simulink model "torqueWalkingMultipleStateCoefficientR2017b"  (Simulink 9.0)
settings: Solver=FixedStepDiscrete  StartTime=0.0  StopTime=Config.t_end  FixedStep=Config.t_step  RelTol=1e-3  EnableMultiTasking=on
InitFcn:
  | cd(fileparts(which(bdroot)));
  | initTorqueWalkingParamInScheme;
StopFcn:
  | cd(fileparts(which(bdroot)));
  | disp_early_termination
undefined symbols (not defined in the file or in its folder): biasVectorConstraint_feet, Config, CONFIG, ConstraintMatrix_feet, DiscIntNeverNeededParam, Gains, ROBOT_DOF, Sat
libraries: WBToolboxLibrary x113, commchan3 x2, simulink x2
(part 2 of 4)

== system torqueWalkingMultipleStateCoefficientR2017b/Robot State and References/Smooth References  ==
  state : Inport
  references_LFoot : Inport  Port=2
  references_RFoot : Inport  Port=3
  references_CoM : Inport  Port=4
  references_rot_task : Inport  Port=5
  references_LHand : Inport  Port=6
  references_RHand : Inport  Port=7
  references_s : Inport  Port=8
  Choose Smoothed or Direct References : Subsystem
  Selector{1..3,5..6} (5 alike) : Selector  NumberOfDimensions=2  InputPortWidth=3  IndexOptions=Index vector (dialog),Index vector (dialog)  Indices=[1:3],1  OutputSizes=1,1
  Selector{8..11} (4 alike) : Selector  NumberOfDimensions=2  InputPortWidth=3  IndexOptions=Index vector (dialog),Index vector (dialog)  Indices=[4:6],[1:3]  OutputSizes=1,1
  Selector4 : Selector  NumberOfDimensions=2  InputPortWidth=3  IndexOptions=Index vector (dialog),Index vector (dialog)  Indices=[1:3],[1:3]  OutputSizes=1,1
  Selector7 : Selector  NumberOfDimensions=2  InputPortWidth=ROBOT_DOF  IndexOptions=Index vector (dialog),Index vector (dialog)  Indices=[1:ROBOT_DOF],1  OutputSizes=1,1
  Smooth Reference Orientations : Subsystem
  Smooth Reference Positions : Subsystem
  pos_vel_acc_CoM_des : Outport
  pose_vel_acc_LFoot_des : Outport  Port=2
  pose_vel_acc_RFoot_des : Outport  Port=3
  orient_vel_acc_rot_task_des : Outport  Port=4
  pose_vel_acc_LHand_des : Outport  Port=5
  pose_vel_acc_RHand_des : Outport  Port=6
  s_sDot_sDDot_ref : Outport  Port=7
  wires:
  references_CoM/1 -> Choose Smoothed or Direct References/7(references_CoM), Selector1/1
  Selector1/1 -> Smooth Reference Positions/1(pos_CoM_des)
  references_LFoot/1 -> Choose Smoothed or Direct References/8(references_LFoot), Selector9/1, Selector2/1
  Selector2/1 -> Smooth Reference Positions/2(pos_LFoot_des)
  references_RFoot/1 -> Selector8/1, Choose Smoothed or Direct References/9(references_RFoot), Selector6/1
  Selector6/1 -> Smooth Reference Positions/3(pos_RFoot_des)
  references_s/1 -> Selector7/1, Choose Smoothed or Direct References/12(references_s)
  Selector7/1 -> Smooth Reference Positions/4(s_des)
  references_rot_task/1 -> Selector4/1, Choose Smoothed or Direct References/13(references_rot_task)
  Selector4/1 -> Smooth Reference Orientations/3(w_R_Rot_task_des)
  Selector8/1 -> Smooth Reference Orientations/2(w_R_RFoot_des)
  Selector9/1 -> Smooth Reference Orientations/1(w_R_LFoot_des)
  Smooth Reference Positions/1(smooth_references_CoM) -> Choose Smoothed or Direct References/1(smooth_references_CoM)
  Smooth Reference Orientations/3(smooth_orient_vel_acc_Rot_task) -> Choose Smoothed or Direct References/16(smooth_references_rot_task)
  Smooth Reference Orientations/2(smooth_orient_vel_acc_RFoot) -> Choose Smoothed or Direct References/15(smooth_orient_vel_acc_RFoot)
  Smooth Reference Orientations/1(smooth_orient_vel_acc_LFoot) -> Choose Smoothed or Direct References/14(smooth_orient_vel_acc_LFoot)
  Choose Smoothed or Direct References/1(pos_vel_acc_CoM_des) -> pos_vel_acc_CoM_des/1
  Choose Smoothed or Direct References/2(pose_vel_acc_LFoot_des) -> pose_vel_acc_LFoot_des/1
  Choose Smoothed or Direct References/7(s_sDot_sDDot_ref) -> s_sDot_sDDot_ref/1
  Choose Smoothed or Direct References/4(orient_vel_acc_rot_task_des) -> orient_vel_acc_rot_task_des/1
  Choose Smoothed or Direct References/3(pose_vel_acc_RFoot_des) -> pose_vel_acc_RFoot_des/1
  state/1 -> Smooth Reference Positions/7(state), Smooth Reference Orientations/6(state)
  Smooth Reference Positions/2(smooth_pos_vel_acc_LFoot) -> Choose Smoothed or Direct References/2(smooth_pos_vel_acc_LFoot)
  Smooth Reference Positions/3(smooth_pos_vel_acc_RFoot) -> Choose Smoothed or Direct References/3(smooth_pos_vel_acc_RFoot)
  Smooth Reference Positions/6(smooth_references_s) -> Choose Smoothed or Direct References/6(smooth_references_s)
  Selector3/1 -> Smooth Reference Positions/5(pos_LHand_des)
  references_LHand/1 -> Selector3/1, Selector11/1, Choose Smoothed or Direct References/10(references_LHand)
  Selector5/1 -> Smooth Reference Positions/6(pos_RHand_des)
  references_RHand/1 -> Selector5/1, Selector10/1, Choose Smoothed or Direct References/11(references_RHand)
  Smooth Reference Positions/4(smooth_pos_vel_acc_LHand) -> Choose Smoothed or Direct References/4(smooth_pos_vel_acc_LHand)
  Smooth Reference Positions/5(smooth_pos_vel_acc_RHand) -> Choose Smoothed or Direct References/5(smooth_pos_vel_acc_RHand)
  Selector11/1 -> Smooth Reference Orientations/4(w_R_LHand_des)
  Selector10/1 -> Smooth Reference Orientations/5(w_R_RHand_des)
  Smooth Reference Orientations/4(smooth_orient_vel_acc_LHand) -> Choose Smoothed or Direct References/17(smooth_orient_vel_acc_LHand)
  Smooth Reference Orientations/5(smooth_orient_vel_acc_RHand) -> Choose Smoothed or Direct References/18(smooth_orient_vel_acc_RHand)
  Choose Smoothed or Direct References/5(pose_vel_acc_LHand_des) -> pose_vel_acc_LHand_des/1
  Choose Smoothed or Direct References/6(pose_vel_acc_RHand_des) -> pose_vel_acc_RHand_des/1

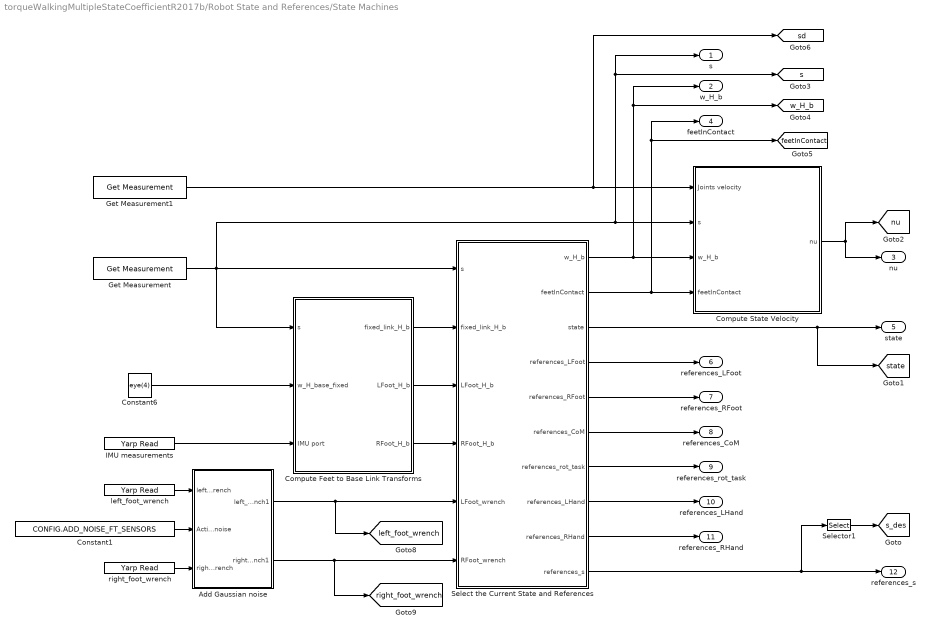
== system torqueWalkingMultipleStateCoefficientR2017b/Robot State and References/State Machines ==
  Add Gaussian noise : Subsystem
  Compute Feet to Base Link Transforms : Subsystem
  Compute State Velocity : Subsystem
  Constant1 : Constant  Value=CONFIG.ADD_NOISE_FT_SENSORS
  Constant6 : Constant  Value=eye(4)
  Get Measurement : WBToolboxLibrary/wholeBodyStates/Get Measurement  measuredType=Joints Position
      settings: SourceProductName=Whole Body Toolbox
  Get Measurement1 : WBToolboxLibrary/wholeBodyStates/Get Measurement  measuredType=Joints Velocity
      settings: SourceProductName=Whole Body Toolbox
  IMU measurements : WBToolboxLibrary/Utilities/Yarp Read  portName=Ports.IMU  signalSize=12  timeout=0.5  blocking=off  timestamp=off  autoconnect=on  errorOnConnection=off
      settings: SourceProductName=Whole Body Toolbox
  Select the Current State and References : Subsystem
  Selector1 : Selector  NumberOfDimensions=2  InputPortWidth=ROBOT_DOF  IndexOptions=Index vector (dialog),Index vector (dialog)  Indices=[1:ROBOT_DOF],1  OutputSizes=1,1
  left_foot_wrench : WBToolboxLibrary/Utilities/Yarp Read  portName=Ports.LEFT_FOOT_EXT_WRENCH  signalSize=6  timeout=0.5  blocking=off  timestamp=off  autoconnect=on  errorOnConnection=on
      settings: SourceProductName=Whole Body Toolbox
  right_foot_wrench : WBToolboxLibrary/Utilities/Yarp Read  portName=Ports.RIGHT_FOOT_EXT_WRENCH  signalSize=6  timeout=0.5  blocking=off  timestamp=off  autoconnect=on  errorOnConnection=on
      settings: SourceProductName=Whole Body Toolbox
  s : Outport
  w_H_b : Outport  Port=2
  nu : Outport  Port=3
  feetInContact : Outport  Port=4
  state : Outport  Port=5
  references_LFoot : Outport  Port=6
  references_RFoot : Outport  Port=7
  references_CoM : Outport  Port=8
  references_rot_task : Outport  Port=9
  references_LHand : Outport  Port=10
  references_RHand : Outport  Port=11
  references_s : Outport  Port=12
  tag scope: feetInContact=global, left_foot_wrench=global, nu=global, right_foot_wrench=global, s=global, s_des=global, sd=global, state=global, w_H_b=global
  wires:
  Get Measurement/1 -> Compute Feet to Base Link Transforms/1(s), Compute State Velocity/2(s), s/1, [s], Select the Current State and References/1(s)
  Constant6/1 -> Compute Feet to Base Link Transforms/2(w_H_base_fixed)
  Compute Feet to Base Link Transforms/1(fixed_link_H_b) -> Select the Current State and References/2(fixed_link_H_b)
  Select the Current State and References/1(w_H_b) -> w_H_b/1, [w_H_b], Compute State Velocity/3(w_H_b)
  Select the Current State and References/2(feetInContact) -> feetInContact/1, [feetInContact], Compute State Velocity/4("feetInContact ")
  Compute State Velocity/1(nu) -> nu/1, [nu]
  Select the Current State and References/3(state) -> [state], state/1
  Select the Current State and References/10(references_s) -> references_s/1, Selector1/1
  Select the Current State and References/6(references_CoM) -> references_CoM/1
  Select the Current State and References/7(references_rot_task) -> references_rot_task/1
  Select the Current State and References/5(references_RFoot) -> references_RFoot/1
  Select the Current State and References/4(references_LFoot) -> references_LFoot/1
  Selector1/1 -> [s_des]
  Compute Feet to Base Link Transforms/2(LFoot_H_b) -> Select the Current State and References/3(LFoot_H_b)
  Compute Feet to Base Link Transforms/3(RFoot_H_b) -> Select the Current State and References/4(RFoot_H_b)
  Select the Current State and References/8(references_LHand) -> references_LHand/1
  Select the Current State and References/9(references_RHand) -> references_RHand/1
  Get Measurement1/1 -> [sd], Compute State Velocity/1(Joints velocity)
  IMU measurements/1 -> Compute Feet to Base Link Transforms/3(IMU port)
  Add Gaussian noise/1(left_foot_wrench1) -> [left_foot_wrench], Select the Current State and References/5(LFoot_wrench)
  Add Gaussian noise/2(right_foot_wrench1) -> [right_foot_wrench], Select the Current State and References/6(RFoot_wrench)
  left_foot_wrench/1 -> Add Gaussian noise/1(left_foot_wrench)
  Constant1/1 -> Add Gaussian noise/2(Activate noise)
  right_foot_wrench/1 -> Add Gaussian noise/3(right_foot_wrench)

== system torqueWalkingMultipleStateCoefficientR2017b/Subsystem/task errors ==
  pos_vel_CoM : Inport
  pos_vel_acc_CoM_des : Inport  Port=2
  orient_vel_rot_rask : Inport  Port=3
  pos_vel_acc_rot_task_des : Inport  Port=4
  pose_vel_LFoot : Inport  Port=5
  pos_vel_acc_LFoot_des : Inport  Port=6
  pose_vel_RFoot : Inport  Port=7
  pos_vel_acc_RFoot_des : Inport  Port=8
  Rotation Error Left Foot : Subsystem
  Rotation Error Left Foot1 : Subsystem
  Rotation Error Rotational Task : Subsystem
  Selector{,2..6} (6 alike) : Selector  NumberOfDimensions=2  InputPortWidth=3  IndexOptions=Index vector (dialog),Index vector (dialog)  Indices=[1:3],1  OutputSizes=1,1
  Selector12 : Selector  NumberOfDimensions=2  InputPortWidth=3  IndexOptions=Index vector (dialog),Index vector (dialog)  Indices=[1:3],[1:3]  OutputSizes=1,1
  Selector13 : Selector  NumberOfDimensions=2  InputPortWidth=3  IndexOptions=Index vector (dialog),Index vector (dialog)  Indices=[1:3],[1:3]  OutputSizes=1,1
  Selector{7..9,15} (4 alike) : Selector  NumberOfDimensions=2  InputPortWidth=3  IndexOptions=Index vector (dialog),Index vector (dialog)  Indices=[4:6],[1:3]  OutputSizes=1,1
  Sum : Sum  Inputs=+-|
  Sum2 : Sum  Inputs=+-|
  Sum3 : Sum  Inputs=+-|
  Vector Concatenate : Concatenate  NumInputs=6
  taskErrors : Outport
  wires:
  Rotation Error Left Foot/1(|1-R^T*RDes|^2) -> Vector Concatenate/4
  Sum3/1 -> Vector Concatenate/5
  Sum2/1 -> Vector Concatenate/3
  Selector6/1 -> Sum3/2
  Selector5/1 -> Sum3/1
  pose_vel_LFoot/1 -> Selector3/1, Selector7/1
  pose_vel_RFoot/1 -> Selector9/1, Selector5/1
  Selector4/1 -> Sum2/2
  Selector/1 -> Sum/1
  Rotation Error Left Foot1/1(|1-R^T*RDes|^2) -> Vector Concatenate/6
  Selector13/1 -> Rotation Error Rotational Task/1(w_R_rot_task)
  Selector12/1 -> Rotation Error Rotational Task/2(w_R_rot_task_des)
  pos_vel_acc_LFoot_des/1 -> Selector15/1, Selector4/1
  Selector15/1 -> Rotation Error Left Foot/2(w_R_RFoot_des)
  Sum/1 -> Vector Concatenate/1
  Rotation Error Rotational Task/1(|1-R^T*RDes|^2) -> Vector Concatenate/2
  Selector8/1 -> Rotation Error Left Foot1/2(w_R_RFoot_des)
  orient_vel_rot_rask/1 -> Selector13/1
  Selector2/1 -> Sum/2
  Selector9/1 -> Rotation Error Left Foot1/1(w_R_RFoot)
  Selector3/1 -> Sum2/1
  pos_vel_acc_rot_task_des/1 -> Selector12/1
  pos_vel_acc_RFoot_des/1 -> Selector8/1, Selector6/1
  pos_vel_CoM/1 -> Selector/1
  Selector7/1 -> Rotation Error Left Foot/1(w_R_RFoot)
  pos_vel_acc_CoM_des/1 -> Selector2/1
  Vector Concatenate/1 -> taskErrors/1

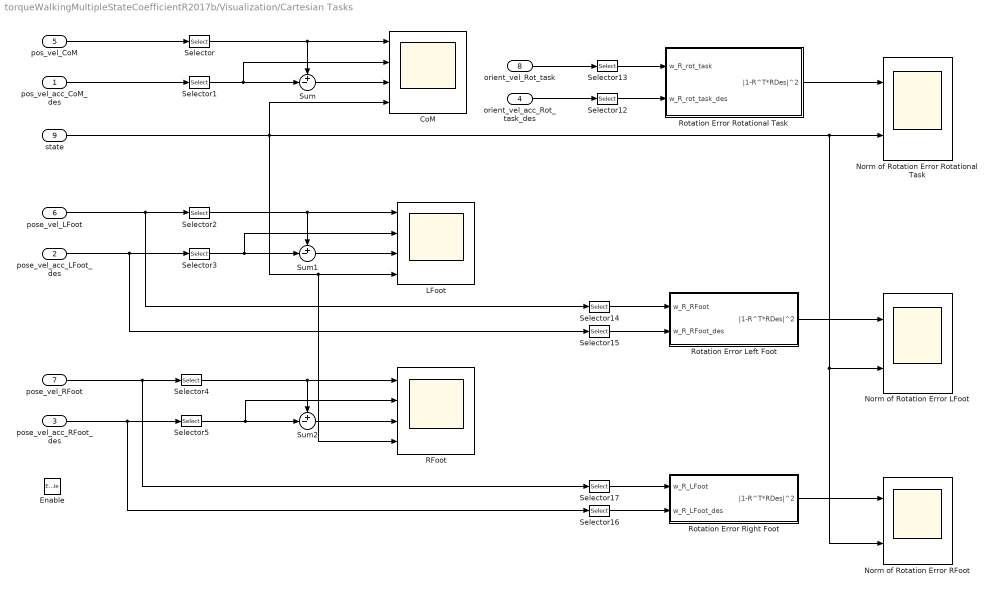
== system torqueWalkingMultipleStateCoefficientR2017b/Visualization/Cartesian Tasks ==
  pos_vel_acc_CoM_des : Inport
  pose_vel_acc_LFoot_des : Inport  Port=2
  pose_vel_acc_RFoot_des : Inport  Port=3
  orient_vel_acc_Rot_task_des : Inport  Port=4
  pos_vel_CoM : Inport  Port=5
  pose_vel_LFoot : Inport  Port=6
  pose_vel_RFoot : Inport  Port=7
  orient_vel_Rot_task : Inport  Port=8
  state : Inport  Port=9
  Enable : EnablePort
  CoM : Scope  NumInputPorts=4
  LFoot : Scope  NumInputPorts=4
  Norm of Rotation Error LFoot : Scope  NumInputPorts=2
  Norm of Rotation Error RFoot : Scope  NumInputPorts=2
  Norm of Rotation Error Rotational Task : Scope  NumInputPorts=2
  RFoot : Scope  NumInputPorts=4
  Rotation Error Left Foot : Subsystem
  Rotation Error Right Foot : Subsystem
  Rotation Error Rotational Task : Subsystem
  Selector{,1..5} (6 alike) : Selector  NumberOfDimensions=2  InputPortWidth=3  IndexOptions=Index vector (dialog),Index vector (dialog)  Indices=[1:3],1  OutputSizes=1,1
  Selector12 : Selector  NumberOfDimensions=2  InputPortWidth=3  IndexOptions=Index vector (dialog),Index vector (dialog)  Indices=[1:3],[1:3]  OutputSizes=1,1
  Selector13 : Selector  NumberOfDimensions=2  InputPortWidth=3  IndexOptions=Index vector (dialog),Index vector (dialog)  Indices=[1:3],[1:3]  OutputSizes=1,1
  Selector{14..17} (4 alike) : Selector  NumberOfDimensions=2  InputPortWidth=3  IndexOptions=Index vector (dialog),Index vector (dialog)  Indices=[4:6],[1:3]  OutputSizes=1,1
  Sum : Sum  Inputs=+-|
  Sum1 : Sum  Inputs=+-|
  Sum2 : Sum  Inputs=+-|
  wires:
  Selector1/1 -> CoM/2, Sum/2
  pos_vel_CoM/1 -> Selector/1
  pos_vel_acc_CoM_des/1 -> Selector1/1
  Selector2/1 -> Sum1/1, LFoot/1
  Selector3/1 -> Sum1/2, LFoot/2
  Selector4/1 -> Sum2/1, RFoot/1
  Selector5/1 -> RFoot/2, Sum2/2
  pose_vel_RFoot/1 -> Selector4/1, Selector17/1
  state/1 -> Norm of Rotation Error RFoot/2, Norm of Rotation Error LFoot/2, Norm of Rotation Error Rotational Task/2, CoM/4, RFoot/4, LFoot/4
  pose_vel_acc_RFoot_des/1 -> Selector5/1, Selector16/1
  pose_vel_LFoot/1 -> Selector2/1, Selector14/1
  Selector12/1 -> Rotation Error Rotational Task/2(w_R_rot_task_des)
  pose_vel_acc_LFoot_des/1 -> Selector15/1, Selector3/1
  orient_vel_acc_Rot_task_des/1 -> Selector12/1
  orient_vel_Rot_task/1 -> Selector13/1
  Selector/1 -> Sum/1, CoM/1
  Sum/1 -> CoM/3
  Sum1/1 -> LFoot/3
  Sum2/1 -> RFoot/3
  Rotation Error Rotational Task/1(|1-R^T*RDes|^2) -> Norm of Rotation Error Rotational Task/1
  Selector13/1 -> Rotation Error Rotational Task/1(w_R_rot_task)
  Rotation Error Left Foot/1(|1-R^T*RDes|^2) -> Norm of Rotation Error LFoot/1
  Selector14/1 -> Rotation Error Left Foot/1(w_R_RFoot)
  Selector15/1 -> Rotation Error Left Foot/2(w_R_RFoot_des)
  Rotation Error Right Foot/1(|1-R^T*RDes|^2) -> Norm of Rotation Error RFoot/1
  Selector16/1 -> Rotation Error Right Foot/2(w_R_LFoot_des)
  Selector17/1 -> Rotation Error Right Foot/1(w_R_LFoot)

== system torqueWalkingMultipleStateCoefficientR2017b/Visualization/Emergency Stop ==
  note: Stop the simulation when the force on each feet is below a threshold (i.e. robot falls)
  F_l_foot : Inport
  F_r_foot : Inport  Port=2
  Enable : EnablePort
  Compare To Constant : simulink/Logic and Bit Operations/Compare To Constant  relop=<=  const=50  OutDataTypeStr=boolean
  Compare To Constant1 : simulink/Logic and Bit Operations/Compare To Constant  relop=<=  const=50  OutDataTypeStr=boolean
  Constant3 : Constant  Value=0  OutDataTypeStr=boolean
  Constant4 : Constant  OutDataTypeStr=boolean
  Logical Operator : Logic  AllPortsSameDT=off  OutDataTypeStr=boolean
  Stop Simulation : Stop
  Switch1 : Switch  Criteria=u2 ~= 0  Threshold=0.5
  To Workspace : ToWorkspace  VariableName=no_force_on_feet  SaveFormat=Timeseries  SampleTime=-1
      settings: MaxDataPoints=1
  select_pose5 : Selector  InputPortWidth=6  IndexOptions=Index vector (dialog)  Indices=[3]  OutputSizes=1
  select_pose6 : Selector  InputPortWidth=6  IndexOptions=Index vector (dialog)  Indices=[3]  OutputSizes=1
  wires:
  F_l_foot/1 -> select_pose5/1
  F_r_foot/1 -> select_pose6/1
  Compare To Constant/1 -> Logical Operator/1
  Compare To Constant1/1 -> Logical Operator/2
  Logical Operator/1 -> Switch1/2
  Switch1/1 -> To Workspace/1, Stop Simulation/1
  Constant4/1 -> Switch1/1
  Constant3/1 -> Switch1/3
  select_pose5/1 -> Compare To Constant/1
  select_pose6/1 -> Compare To Constant1/1

== system torqueWalkingMultipleStateCoefficientR2017b/Visualization/Emergency Stop1 ==
  exitFlagQP : Inport
  Enable : EnablePort
  Constant : Constant  Value=2
  Constant1 : Constant  Value=0  OutDataTypeStr=boolean
  Constant2 : Constant  OutDataTypeStr=boolean
  Stop Simulation : Stop
  Sum : Sum  Inputs=|++
  Switch : Switch  Criteria=u2 > Threshold  Threshold=0.1
  To Workspace : ToWorkspace  VariableName=exitFlagQP_unsuccessful  SaveFormat=Timeseries  SampleTime=-1
      settings: MaxDataPoints=1
  wires:
  exitFlagQP/1 -> Sum/1
  Sum/1 -> Switch/2
  Constant/1 -> Sum/2
  Constant1/1 -> Switch/1
  Constant2/1 -> Switch/3
  Switch/1 -> To Workspace/1, Stop Simulation/1

== system torqueWalkingMultipleStateCoefficientR2017b/Visualization/Emergency Stop2 ==
  note: Stop the simulation when the ZMP goes out of the support polygon
  ZMP : Inport
  support_polygon : Inport  Port=2
  Enable : EnablePort
  Constant3 : Constant  Value=0  OutDataTypeStr=boolean
  Constant4 : Constant  OutDataTypeStr=boolean
  Logical Operator : Logic  Operator=OR  AllPortsSameDT=off  OutDataTypeStr=boolean
  Logical Operator1 : Logic  Operator=OR  AllPortsSameDT=off  OutDataTypeStr=boolean
  Logical Operator2 : Logic  Operator=OR  AllPortsSameDT=off  OutDataTypeStr=boolean
  Logical Operator3 : Logic  Inputs=3  AllPortsSameDT=off  OutDataTypeStr=boolean
  Memory{,1..3} (4 alike) : Memory
  Relational Operator : RelationalOperator  Operator=<  OutDataTypeStr=boolean  RndMeth=Simplest
  Relational Operator1 : RelationalOperator  Operator=>  OutDataTypeStr=boolean  RndMeth=Simplest
  Relational Operator2 : RelationalOperator  Operator=<  OutDataTypeStr=boolean  RndMeth=Simplest
  Relational Operator3 : RelationalOperator  Operator=>  OutDataTypeStr=boolean  RndMeth=Simplest
  Relational Operator4 : RelationalOperator  Operator=<  OutDataTypeStr=boolean  RndMeth=Simplest
  Relational Operator5 : RelationalOperator  Operator=>  OutDataTypeStr=boolean  RndMeth=Simplest
  Stop Simulation : Stop
  Sum of Elements : Sum  Inputs=+
  Switch1 : Switch  Criteria=u2 ~= 0  Threshold=0.5
  To Workspace : ToWorkspace  VariableName=ZMP_out_of_bounds  SaveFormat=Timeseries  SampleTime=-1
      settings: MaxDataPoints=1
  select_pose1 : Selector  NumberOfDimensions=2  InputPortWidth=6  IndexOptions=Index vector (dialog),Index vector (dialog)  Indices=[1 2],2  OutputSizes=1,1
  select_pose2 : Selector  NumberOfDimensions=2  InputPortWidth=6  IndexOptions=Index vector (dialog),Index vector (dialog)  Indices=[1 2],2  OutputSizes=1,1
  select_pose3 : Selector  NumberOfDimensions=2  InputPortWidth=6  IndexOptions=Index vector (dialog),Index vector (dialog)  Indices=[1 2],1  OutputSizes=1,1
  select_pose4 : Selector  NumberOfDimensions=2  InputPortWidth=6  IndexOptions=Index vector (dialog),Index vector (dialog)  Indices=[1 2],2  OutputSizes=1,1
  select_pose5 : Selector  NumberOfDimensions=2  InputPortWidth=6  IndexOptions=Index vector (dialog),Index vector (dialog)  Indices=[1 2],1  OutputSizes=1,1
  select_pose6 : Selector  NumberOfDimensions=2  InputPortWidth=6  IndexOptions=Index vector (dialog),Index vector (dialog)  Indices=[1 2],1  OutputSizes=1,1
  wires:
  Constant3/1 -> Switch1/3
  Constant4/1 -> Switch1/1
  Switch1/1 -> To Workspace/1, Stop Simulation/1
  Sum of Elements/1 -> Switch1/2
  select_pose6/1 -> Relational Operator/2
  select_pose1/1 -> Relational Operator1/2
  Relational Operator/1 -> Logical Operator/1
  Relational Operator1/1 -> Logical Operator/2
  Logical Operator/1 -> Logical Operator3/1
  support_polygon/1 -> Memory/1, select_pose1/1, select_pose6/1
  ZMP/1 -> Memory1/1, Relational Operator1/1, Relational Operator/1
  Logical Operator1/1 -> Logical Operator3/2
  select_pose3/1 -> Relational Operator2/2
  Relational Operator3/1 -> Logical Operator1/2
  Relational Operator2/1 -> Logical Operator1/1
  select_pose2/1 -> Relational Operator3/2
  Memory/1 -> Memory2/1, select_pose2/1, select_pose3/1
  Memory2/1 -> select_pose4/1, select_pose5/1
  Memory3/1 -> Relational Operator5/1, Relational Operator4/1
  select_pose4/1 -> Relational Operator5/2
  Memory1/1 -> Memory3/1, Relational Operator3/1, Relational Operator2/1
  select_pose5/1 -> Relational Operator4/2
  Relational Operator4/1 -> Logical Operator2/1
  Relational Operator5/1 -> Logical Operator2/2
  Logical Operator2/1 -> Logical Operator3/3
  Logical Operator3/1 -> Sum of Elements/1

== system torqueWalkingMultipleStateCoefficientR2017b/Visualization/External wrench  applied ==
  Constant : Constant  Value=CONFIG.APPLY_EXTERNAL_WRENCH
  don't check ZMP : Outport
  wires:
  Constant/1 -> don't check ZMP/1

== system torqueWalkingMultipleStateCoefficientR2017b/Visualization/Forces and Torques ==
  tau measured : Inport
  tau desired : Inport  Port=2
  f LFoot desired : Inport  Port=3
  f RFoot desired : Inport  Port=4
  exitFlag QP : Inport  Port=5
  f LFoot : Inport  Port=6
  f RFoot : Inport  Port=7
  state : Inport  Port=8
  Enable : EnablePort
  Demux{1..4} (4 alike) : Demux  Outputs=[3;3]
  DoFs converter : WBToolboxLibrary/Utilities/DoFs converter  yarp2WBIOption=From YARP to WBI
      settings: SourceProductName=Whole Body Toolbox
  DoFs converter1 : WBToolboxLibrary/Utilities/DoFs converter  yarp2WBIOption=From YARP to WBI
      settings: SourceProductName=Whole Body Toolbox
  DoFs converter2 : WBToolboxLibrary/Utilities/DoFs converter  yarp2WBIOption=From YARP to WBI
      settings: SourceProductName=Whole Body Toolbox
  QP status : Scope  NumInputPorts=2
  Sum : Sum  Inputs=+-|
  Sum1 : Sum  Inputs=|+-
  Sum2 : Sum  Inputs=+-|
  Sum3 : Sum  Inputs=|+-
  Sum4 : Sum  Inputs=+-|
  desired torque : Scope  NumInputPorts=6
  forces Left Foot : Scope  NumInputPorts=4
  forces Right Foot : Scope  NumInputPorts=4
  measured torque : Scope  NumInputPorts=6
  moments Left Foot : Scope  NumInputPorts=4
  moments Right Foot : Scope  NumInputPorts=4
  torque error : Scope  NumInputPorts=6
  wires:
  Sum2/1 -> moments Left Foot/3  "moments measured left foot"
  state/1 -> QP status/2, torque error/6, desired torque/6, forces Right Foot/4, moments Right Foot/4, forces Left Foot/4, moments Left Foot/4, measured torque/6
  DoFs converter1/2 -> desired torque/2  "left_arm"
  Demux4/1 -> forces Left Foot/2, Sum1/2  "force desired left foot"
  DoFs converter2/1 -> torque error/1  "torso"
  DoFs converter1/4 -> desired torque/4  "left_leg"
  Demux4/2 -> moments Left Foot/2, Sum2/2  "moments measured left foot"
  DoFs converter/1 -> measured torque/1  "torso"
  DoFs converter2/3 -> torque error/3  "right_arm"
  f RFoot desired/1 -> Demux3/1
  DoFs converter1/1 -> desired torque/1  "torso"
  Sum4/1 -> moments Right Foot/3  "moments measured right foot"
  tau desired/1 -> Sum/2, DoFs converter1/1
  Demux2/1 -> forces Right Foot/1, Sum3/1  "force measured right foot"
  DoFs converter2/2 -> torque error/2  "left_arm"
  Sum3/1 -> forces Right Foot/3  "force error right foot"
  DoFs converter/5 -> measured torque/5  "right_leg"
  DoFs converter2/5 -> torque error/5  "right_leg"
  exitFlag QP/1 -> QP status/1
  f LFoot/1 -> Demux1/1  "wL_WBDT"
  DoFs converter1/3 -> desired torque/3  "right_arm"
  Demux3/1 -> forces Right Foot/2, Sum3/2  "force desired right foot"
  f LFoot desired/1 -> Demux4/1
  Sum1/1 -> forces Left Foot/3  "force error left foot"
  tau measured/1 -> Sum/1, DoFs converter/1
  DoFs converter1/5 -> desired torque/5  "right_leg"
  DoFs converter/2 -> measured torque/2  "left_arm"
  DoFs converter/3 -> measured torque/3  "right_arm"
  Demux3/2 -> moments Right Foot/2, Sum4/2  "moments measured right foot"
  Sum/1 -> DoFs converter2/1
  Demux1/1 -> forces Left Foot/1, Sum1/1  "force measured left foot"
  DoFs converter/4 -> measured torque/4  "left_leg"
  Demux1/2 -> moments Left Foot/1, Sum2/1  "moments measured left foot"
  f RFoot/1 -> Demux2/1  "wR_WBDT"
  DoFs converter2/4 -> torque error/4  "left_leg"
  Demux2/2 -> moments Right Foot/1, Sum4/1  "moments measured right foot"

== system torqueWalkingMultipleStateCoefficientR2017b/Visualization/Gain Scheduling ==
  Kp_CoM : Inport
  Kd_CoM : Inport  Port=2
  Kp_LFoot : Inport  Port=3
  Kd_LFoot : Inport  Port=4
  Kp_RFoot : Inport  Port=5
  Kd_RFoot : Inport  Port=6
  Kp_rot_task : Inport  Port=7
  Kd_rot_task : Inport  Port=8
  impedances : Inport  Port=9
  dampings : Inport  Port=10
  state : Inport  Port=11
  Enable : EnablePort
  DoFs converter1 : WBToolboxLibrary/Utilities/DoFs converter  yarp2WBIOption=From YARP to WBI
      settings: SourceProductName=Whole Body Toolbox
  DoFs converter4 : WBToolboxLibrary/Utilities/DoFs converter  yarp2WBIOption=From YARP to WBI
      settings: SourceProductName=Whole Body Toolbox
  joint position gains : Scope  NumInputPorts=6
  joint velocity gains : Scope  NumInputPorts=6
  orient gains rot task : Scope  NumInputPorts=2
  pos gains CoM : Scope  NumInputPorts=2
  pose gains LFoot : Scope  NumInputPorts=2
  pose gains RFoot : Scope  NumInputPorts=2
  vel gains CoM : Scope  NumInputPorts=2
  vel gains LFoot : Scope  NumInputPorts=2
  vel gains RFoot : Scope  NumInputPorts=2
  vel gains rot task : Scope  NumInputPorts=2
  wires:
  Kp_CoM/1 -> pos gains CoM/1
  Kp_LFoot/1 -> pose gains LFoot/1
  Kp_RFoot/1 -> pose gains RFoot/1
  Kp_rot_task/1 -> orient gains rot task/1
  state/1 -> vel gains LFoot/2, pose gains LFoot/2, vel gains CoM/2, vel gains rot task/2, orient gains rot task/2, vel gains RFoot/2, joint velocity gains/6, joint position gains/6, pose gains RFoot/2, pos gains CoM/2
  Kd_CoM/1 -> vel gains CoM/1
  Kd_LFoot/1 -> vel gains LFoot/1
  Kd_RFoot/1 -> vel gains RFoot/1
  Kd_rot_task/1 -> vel gains rot task/1
  DoFs converter4/2 -> joint position gains/2  "left_arm"
  DoFs converter4/1 -> joint position gains/1  "torso"
  DoFs converter4/4 -> joint position gains/4  "left_leg"
  DoFs converter4/3 -> joint position gains/3  "right_arm"
  DoFs converter4/5 -> joint position gains/5  "right_leg"
  DoFs converter1/2 -> joint velocity gains/2  "left_arm"
  DoFs converter1/1 -> joint velocity gains/1  "torso"
  DoFs converter1/4 -> joint velocity gains/4  "left_leg"
  DoFs converter1/3 -> joint velocity gains/3  "right_arm"
  DoFs converter1/5 -> joint velocity gains/5  "right_leg"
  impedances/1 -> DoFs converter4/1
  dampings/1 -> DoFs converter1/1

== system torqueWalkingMultipleStateCoefficientR2017b/Visualization/Joints and Floating Base State ==
  s : Inport
  w_H_b : Inport  Port=2
  nu : Inport  Port=3
  state : Inport  Port=4
  s_des : Inport  Port=5
  feetInContact : Inport  Port=6
  Enable : EnablePort
  DoFs converter{,1..3} (4 alike) : WBToolboxLibrary/Utilities/DoFs converter  yarp2WBIOption=From YARP to WBI
      settings: SourceProductName=Whole Body Toolbox
  Gain : Gain  Gain=180/pi
  Gain1 : Gain  Gain=180/pi
  Gain2 : Gain  Gain=180/pi
  Selector : Selector  NumberOfDimensions=2  InputPortWidth=3  IndexOptions=Index vector (dialog),Index vector (dialog)  Indices=[1:3],4  OutputSizes=1,1
  Selector1 : Selector  InputPortWidth=ROBOT_DOF+6  IndexOptions=Index vector (dialog)  Indices=[1:6]  OutputSizes=1
  Selector2 : Selector  InputPortWidth=ROBOT_DOF+6  IndexOptions=Index vector (dialog)  Indices=[7:ROBOT_DOF+6]  OutputSizes=1
  Sum : Sum  Inputs=+-|
  base position : Scope  NumInputPorts=2
  base velocity : Scope  NumInputPorts=2
  desired joint pos : Scope  NumInputPorts=6
  feet in contact : Scope  NumInputPorts=2
  joint error : Scope  NumInputPorts=6
  joint velocity : Scope  NumInputPorts=6
  measured joint pos : Scope  NumInputPorts=6
  wires:
  DoFs converter1/2 -> desired joint pos/2  "left_arm"
  DoFs converter/5 -> measured joint pos/5  "right_leg"
  DoFs converter2/1 -> joint error/1  "torso"
  DoFs converter/4 -> measured joint pos/4  "left_leg"
  DoFs converter/2 -> measured joint pos/2  "left_arm"
  s/1 -> Gain/1
  DoFs converter1/1 -> desired joint pos/1  "torso"
  DoFs converter1/4 -> desired joint pos/4  "left_leg"
  DoFs converter1/3 -> desired joint pos/3  "right_arm"
  DoFs converter/3 -> measured joint pos/3  "right_arm"
  DoFs converter2/5 -> joint error/5  "right_leg"
  DoFs converter2/2 -> joint error/2  "left_arm"
  DoFs converter/1 -> measured joint pos/1  "torso"
  s_des/1 -> Gain1/1
  DoFs converter1/5 -> desired joint pos/5  "right_leg"
  DoFs converter2/4 -> joint error/4  "left_leg"
  DoFs converter2/3 -> joint error/3  "right_arm"
  DoFs converter3/5 -> joint velocity/5  "right_leg"
  DoFs converter3/1 -> joint velocity/1  "torso"
  DoFs converter3/4 -> joint velocity/4  "left_leg"
  DoFs converter3/3 -> joint velocity/3  "right_arm"
  DoFs converter3/2 -> joint velocity/2  "left_arm"
  nu/1 -> Selector2/1, Selector1/1
  w_H_b/1 -> Selector/1
  Gain/1 -> Sum/1, DoFs converter/1
  Gain1/1 -> Sum/2, DoFs converter1/1
  Gain2/1 -> DoFs converter3/1
  Selector/1 -> base position/1
  Selector2/1 -> Gain2/1
  state/1 -> measured joint pos/6, joint velocity/6, base velocity/2, feet in contact/2, base position/2, joint error/6, desired joint pos/6
  Selector1/1 -> base velocity/1
  feetInContact/1 -> feet in contact/1
  Sum/1 -> DoFs converter2/1

== system torqueWalkingMultipleStateCoefficientR2017b/Visualization/Orientation Tasks References ==
  w_R_LFoot_des : Inport
  w_R_RFoot_des : Inport  Port=2
  w_R_rot_task_des : Inport  Port=3
  w_R_LFoot : Inport  Port=4
  w_R_RFoot : Inport  Port=5
  w_R_rot_task : Inport  Port=6
  omegaDot_LFoot : Inport  Port=7
  omegaDot_RFoot : Inport  Port=8
  omegaDot_rot_task : Inport  Port=9
  omega_rot_task : Inport  Port=10
  omega_RFoot : Inport  Port=11
  omega_LFoot : Inport  Port=12
  Enable : EnablePort
  LFoot omega : Scope
  LFoot omegaDot : Scope
  Norm of Rotation Error LFoot : Scope
  Norm of Rotation Error RFoot : Scope
  Norm of Rotation Error rot_task : Scope
  RFoot omega : Scope
  RFoot omegaDot : Scope
  Rotation Error Left Foot : Subsystem
  Rotation Error Right Foot : Subsystem
  Rotation Error Rotational Task : Subsystem
  rot_task omega : Scope
  rot_task omegaDot : Scope
  wires:
  omega_rot_task/1 -> rot_task omega/1
  omega_RFoot/1 -> RFoot omega/1
  omega_LFoot/1 -> LFoot omega/1
  omegaDot_LFoot/1 -> LFoot omegaDot/1
  omegaDot_RFoot/1 -> RFoot omegaDot/1
  omegaDot_rot_task/1 -> rot_task omegaDot/1
  Rotation Error Left Foot/1(|1-R^T*RDes|^2) -> Norm of Rotation Error LFoot/1
  w_R_LFoot/1 -> Rotation Error Left Foot/1(w_R_LFoot)
  w_R_LFoot_des/1 -> Rotation Error Left Foot/2(w_R_LFoot_des)
  Rotation Error Right Foot/1(|1-R^T*RDes|^2) -> Norm of Rotation Error RFoot/1
  w_R_RFoot/1 -> Rotation Error Right Foot/1(w_R_RFoot)
  w_R_RFoot_des/1 -> Rotation Error Right Foot/2(w_R_RFoot_des)
  Rotation Error Rotational Task/1(|1-R^T*RDes|^2) -> Norm of Rotation Error rot_task/1
  w_R_rot_task/1 -> Rotation Error Rotational Task/1(w_R_rot_task)
  w_R_rot_task_des/1 -> Rotation Error Rotational Task/2(w_R_rot_task_des)

== system torqueWalkingMultipleStateCoefficientR2017b/synchronizer/GAZEBO_SYNCHRONIZER ==
  Enable : EnablePort
  Simulator Synchronizer : WBToolboxLibrary/Utilities/Simulator Synchronizer  period=Config.t_step  serverPortName='/clock/rpc'  clientPortName='/WBT_synchronizer/rpc:o'
      settings: SourceProductName=Whole Body Toolbox

== system torqueWalkingMultipleStateCoefficientR2017b/synchronizer/REAL_TIME_SYNC ==
  Enable : EnablePort
  Real Time Synchronizer : WBToolboxLibrary/Utilities/Real Time Synchronizer  period=Config.t_step
      settings: SourceProductName=Whole Body Toolbox

== system torqueWalkingMultipleStateCoefficientR2017b/Dynamics and Kinematics/Compute Dynamic and Kinematic Quantities/Jacobians and JDot_nu ==
  s : Inport
  nu_b : Inport  Port=2
  sDot : Inport  Port=3
  w_H_b : Inport  Port=4
  DotJ Nu CoM : WBToolboxLibrary/wholeBodyModel/Jacobians/DotJ Nu  frameName=Frames.COM
      settings: SourceProductName=Whole Body Toolbox
  DotJ Nu LFoot : WBToolboxLibrary/wholeBodyModel/Jacobians/DotJ Nu  frameName=Frames.LEFT_FOOT
      settings: SourceProductName=Whole Body Toolbox
  DotJ Nu LHand : WBToolboxLibrary/wholeBodyModel/Jacobians/DotJ Nu  frameName=Frames.LEFT_HAND
      settings: SourceProductName=Whole Body Toolbox
  DotJ Nu RFoot : WBToolboxLibrary/wholeBodyModel/Jacobians/DotJ Nu  frameName=Frames.RIGHT_FOOT
      settings: SourceProductName=Whole Body Toolbox
  DotJ Nu RHand : WBToolboxLibrary/wholeBodyModel/Jacobians/DotJ Nu  frameName=Frames.RIGHT_HAND
      settings: SourceProductName=Whole Body Toolbox
  DotJ Nu rotational task : WBToolboxLibrary/wholeBodyModel/Jacobians/DotJ Nu  frameName=Frames.ROT_TASK_LINK
      settings: SourceProductName=Whole Body Toolbox
  Jacobian CoM : WBToolboxLibrary/wholeBodyModel/Jacobians/Jacobian  frameName=Frames.COM
      settings: SourceProductName=Whole Body Toolbox
  Jacobian LFoot : WBToolboxLibrary/wholeBodyModel/Jacobians/Jacobian  frameName=Frames.LEFT_FOOT
      settings: SourceProductName=Whole Body Toolbox
  Jacobian LHand : WBToolboxLibrary/wholeBodyModel/Jacobians/Jacobian  frameName=Frames.LEFT_HAND
      settings: SourceProductName=Whole Body Toolbox
  Jacobian RFoot : WBToolboxLibrary/wholeBodyModel/Jacobians/Jacobian  frameName=Frames.RIGHT_FOOT
      settings: SourceProductName=Whole Body Toolbox
  Jacobian RHand : WBToolboxLibrary/wholeBodyModel/Jacobians/Jacobian  frameName=Frames.RIGHT_HAND
      settings: SourceProductName=Whole Body Toolbox
  Jacobian rotational task : WBToolboxLibrary/wholeBodyModel/Jacobians/Jacobian  frameName=Frames.ROT_TASK_LINK
      settings: SourceProductName=Whole Body Toolbox
  J_LFoot : Outport
  J_RFoot : Outport  Port=2
  J_CoM : Outport  Port=3
  J_rot_task : Outport  Port=4
  J_LHand : Outport  Port=5
  J_RHand : Outport  Port=6
  JDot_nu_LFoot : Outport  Port=7
  JDot_nu_RFoot : Outport  Port=8
  JDot_nu_CoM : Outport  Port=9
  JDot_nu_rot_task : Outport  Port=10
  JDot_nu_LHand : Outport  Port=11
  JDot_nu_RHand : Outport  Port=12
  wires:
  Jacobian CoM/1 -> J_CoM/1
  Jacobian rotational task/1 -> J_rot_task/1
  Jacobian LFoot/1 -> J_LFoot/1
  Jacobian RFoot/1 -> J_RFoot/1
  w_H_b/1 -> Jacobian RHand/1, Jacobian LHand/1, Jacobian RFoot/1, Jacobian LFoot/1, DotJ Nu RHand/1, DotJ Nu LHand/1, DotJ Nu RFoot/1, DotJ Nu LFoot/1, DotJ Nu rotational task/1, DotJ Nu CoM/1, Jacobian CoM/1, Jacobian rotational task/1
  sDot/1 -> DotJ Nu RFoot/4, DotJ Nu RHand/4, DotJ Nu LHand/4, DotJ Nu LFoot/4, DotJ Nu rotational task/4, DotJ Nu CoM/4
  nu_b/1 -> DotJ Nu CoM/3, DotJ Nu RHand/3, DotJ Nu LHand/3, DotJ Nu RFoot/3, DotJ Nu LFoot/3, DotJ Nu rotational task/3
  s/1 -> Jacobian RHand/2, Jacobian LHand/2, DotJ Nu RHand/2, DotJ Nu LHand/2, DotJ Nu RFoot/2, DotJ Nu LFoot/2, DotJ Nu rotational task/2, DotJ Nu CoM/2, Jacobian RFoot/2, Jacobian CoM/2, Jacobian rotational task/2, Jacobian LFoot/2
  DotJ Nu RFoot/1 -> JDot_nu_RFoot/1
  DotJ Nu LFoot/1 -> JDot_nu_LFoot/1
  DotJ Nu rotational task/1 -> JDot_nu_rot_task/1
  DotJ Nu CoM/1 -> JDot_nu_CoM/1
  Jacobian RHand/1 -> J_RHand/1
  Jacobian LHand/1 -> J_LHand/1
  DotJ Nu LHand/1 -> JDot_nu_LHand/1
  DotJ Nu RHand/1 -> JDot_nu_RHand/1

== system torqueWalkingMultipleStateCoefficientR2017b/Dynamics and Kinematics/Compute Dynamic and Kinematic Quantities/Mass Matrix and Bias Forces ==
  s : Inport
  nu_b : Inport  Port=2
  sDot : Inport  Port=3
  w_H_b : Inport  Port=4
  Add motors reflected inertias : Subsystem
  Get Bias Forces : WBToolboxLibrary/wholeBodyModel/Dynamics/Get Bias Forces
      settings: SourceProductName=Whole Body Toolbox
  Mass Matrix : WBToolboxLibrary/wholeBodyModel/Dynamics/Mass Matrix
      settings: SourceProductName=Whole Body Toolbox
  h(q,nu) : Outport
  M(q) : Outport  Port=2
  wires:
  w_H_b/1 -> Mass Matrix/1, Get Bias Forces/1
  s/1 -> Mass Matrix/2, Get Bias Forces/2
  sDot/1 -> Get Bias Forces/4
  nu_b/1 -> Get Bias Forces/3
  Get Bias Forces/1 -> h(q,nu)/1
  Mass Matrix/1 -> Add motors reflected inertias/1(M)
  Add motors reflected inertias/1(M_with_motor_inertia) -> M(q)/1

== system torqueWalkingMultipleStateCoefficientR2017b/Dynamics and Kinematics/Initial Conditions/Compute world to base transform ==
  s : Inport
  Constant : Constant  Value=Config.LFoot_in_contact_at0
  Constant6 : Constant  Value=eye(4)
  "Inv\\*  " : Product  Inputs=/*  Multiplication=Matrix(*)
  Switch6 : Switch  Criteria=u2 > Threshold
  left foot : WBToolboxLibrary/wholeBodyModel/Kinematics/Forward Kinematics  frameName=Frames.LEFT_FOOT
      settings: SourceProductName=Whole Body Toolbox
  left foot1 : WBToolboxLibrary/wholeBodyModel/Kinematics/Forward Kinematics  frameName=Frames.RIGHT_FOOT
      settings: SourceProductName=Whole Body Toolbox
  root_link : WBToolboxLibrary/wholeBodyModel/Kinematics/Forward Kinematics  frameName='root_link'
      settings: SourceProductName=Whole Body Toolbox
  w_H_b : Outport
  wires:
  Constant/1 -> Switch6/2
  left foot1/1 -> Switch6/1
  s/1 -> root_link/2, left foot/2, left foot1/2
  left foot/1 -> Switch6/3
  "Inv\\*  "/1 -> w_H_b/1
  Constant6/1 -> left foot/1, root_link/1, left foot1/1
  Switch6/1 -> "Inv\\*  "/1
  root_link/1 -> "Inv\\*  "/2

== system torqueWalkingMultipleStateCoefficientR2017b/Dynamics and Kinematics/Initial Conditions/compute state velocity ==
  s : Inport
  w_H_b : Inport  Port=2
  "feetInContact " : Inport  Port=3
  sDot : Inport  Port=4
  Compute Base Velocity : MATLAB Function  TreatAsAtomicUnit=on
  Feet Jacobians : Subsystem
  Mux : Mux  Inputs=2
  nu : Outport
  wires:
  w_H_b/1 -> Feet Jacobians/2(w_H_b)
  "feetInContact "/1 -> Compute Base Velocity/3(feetInContact)
  Mux/1 -> nu/1
  s/1 -> Feet Jacobians/1(s)
  Compute Base Velocity/1(nu_b) -> Mux/1
  sDot/1 -> Mux/2, Compute Base Velocity/4(sDot)
  Feet Jacobians/1(J_LFoot) -> Compute Base Velocity/1(J_LeftFoot)
  Feet Jacobians/2(J_RFoot) -> Compute Base Velocity/2(J_RightFoot)

== system torqueWalkingMultipleStateCoefficientR2017b/Dynamics and Kinematics/Inverse Kinematics/ComputeTasksPoseAndVelocity ==
  J_LFoot : Inport
  J_RFoot : Inport  Port=2
  J_CoM : Inport  Port=3
  J_rot_task : Inport  Port=4
  J_LHand : Inport  Port=5
  J_RHand : Inport  Port=6
  qj : Inport  Port=7
  w_H_b : Inport  Port=8
  nu : Inport  Port=9
  Compose Task Pose and Velocity : MATLAB Function  TreatAsAtomicUnit=on
  Product{,1..5} (6 alike) : Product  Multiplication=Matrix(*)
  Task position and orientation : Subsystem
  pose_vel_LFoot : Outport
  pose_vel_RFoot : Outport  Port=2
  pos_vel_CoM : Outport  Port=3
  orient_vel_rot_task : Outport  Port=4
  pose_vel_LHand : Outport  Port=5
  pose_vel_RHand : Outport  Port=6
  wires:
  Compose Task Pose and Velocity/2(pose_vel_RFoot) -> pose_vel_RFoot/1
  Compose Task Pose and Velocity/1(pose_vel_LFoot) -> pose_vel_LFoot/1
  Compose Task Pose and Velocity/3(pos_vel_CoM) -> pos_vel_CoM/1
  Compose Task Pose and Velocity/4(orient_vel_rot_task) -> orient_vel_rot_task/1
  nu/1 -> Product5/2, Product4/2, Product/2, Product1/2, Product2/2, Product3/2
  J_rot_task/1 -> Product3/1
  Product/1 -> Compose Task Pose and Velocity/3(vel_CoM)
  Product1/1 -> Compose Task Pose and Velocity/1(vel_LFoot)
  Product2/1 -> Compose Task Pose and Velocity/2(vel_RFoot)
  Product3/1 -> Compose Task Pose and Velocity/4(vel_rot_task)
  qj/1 -> Task position and orientation/1(s)
  w_H_b/1 -> Task position and orientation/2(w_H_b)
  Task position and orientation/3(w_H_CoM) -> Compose Task Pose and Velocity/9(w_H_CoM)
  Task position and orientation/1(w_H_l_sole) -> Compose Task Pose and Velocity/7(w_H_l_sole)
  Task position and orientation/2(w_H_r_sole) -> Compose Task Pose and Velocity/8(w_H_r_sole)
  Task position and orientation/4(w_H_rot_task) -> Compose Task Pose and Velocity/10(w_H_rot_task)
  J_LFoot/1 -> Product1/1
  J_CoM/1 -> Product/1
  J_RFoot/1 -> Product2/1
  J_LHand/1 -> Product4/1
  J_RHand/1 -> Product5/1
  Product4/1 -> Compose Task Pose and Velocity/5(vel_LHand)
  Product5/1 -> Compose Task Pose and Velocity/6(vel_RHand)
  Task position and orientation/5(w_H_l_hand) -> Compose Task Pose and Velocity/11(w_H_l_hand)
  Task position and orientation/6(w_H_r_hand) -> Compose Task Pose and Velocity/12(w_H_r_hand)
  Compose Task Pose and Velocity/5(pose_vel_LHand) -> pose_vel_LHand/1
  Compose Task Pose and Velocity/6(pose_vel_RHand) -> pose_vel_RHand/1

== system torqueWalkingMultipleStateCoefficientR2017b/Dynamics and Kinematics/Inverse Kinematics/Jacobians and JDot_nu ==
  s : Inport
  w_H_b : Inport  Port=2
  nu_b : Inport  Port=3
  sDot : Inport  Port=4
  DotJ Nu CoM : WBToolboxLibrary/wholeBodyModel/Jacobians/DotJ Nu  frameName=Frames.COM
      settings: SourceProductName=Whole Body Toolbox
  DotJ Nu LFoot : WBToolboxLibrary/wholeBodyModel/Jacobians/DotJ Nu  frameName=Frames.LEFT_FOOT
      settings: SourceProductName=Whole Body Toolbox
  DotJ Nu LHand : WBToolboxLibrary/wholeBodyModel/Jacobians/DotJ Nu  frameName=Frames.LEFT_FOOT
      settings: SourceProductName=Whole Body Toolbox
  DotJ Nu RHand : WBToolboxLibrary/wholeBodyModel/Jacobians/DotJ Nu  frameName=Frames.RIGHT_FOOT
      settings: SourceProductName=Whole Body Toolbox
  DotJ Nu Rfoot : WBToolboxLibrary/wholeBodyModel/Jacobians/DotJ Nu  frameName=Frames.RIGHT_FOOT
      settings: SourceProductName=Whole Body Toolbox
  DotJ Nu rotational task : WBToolboxLibrary/wholeBodyModel/Jacobians/DotJ Nu  frameName=Frames.ROT_TASK_LINK
      settings: SourceProductName=Whole Body Toolbox
  Jacobian CoM : WBToolboxLibrary/wholeBodyModel/Jacobians/Jacobian  frameName=Frames.COM
      settings: SourceProductName=Whole Body Toolbox
  Jacobian LFoot : WBToolboxLibrary/wholeBodyModel/Jacobians/Jacobian  frameName=Frames.LEFT_FOOT
      settings: SourceProductName=Whole Body Toolbox
  Jacobian LFoot1 : WBToolboxLibrary/wholeBodyModel/Jacobians/Jacobian  frameName=Frames.LEFT_HAND
      settings: SourceProductName=Whole Body Toolbox
  Jacobian RFoot : WBToolboxLibrary/wholeBodyModel/Jacobians/Jacobian  frameName=Frames.RIGHT_FOOT
      settings: SourceProductName=Whole Body Toolbox
  Jacobian RFoot1 : WBToolboxLibrary/wholeBodyModel/Jacobians/Jacobian  frameName=Frames.RIGHT_HAND
      settings: SourceProductName=Whole Body Toolbox
  Jacobian rotational task : WBToolboxLibrary/wholeBodyModel/Jacobians/Jacobian  frameName=Frames.ROT_TASK_LINK
      settings: SourceProductName=Whole Body Toolbox
  J_LFoot : Outport
  J_RFoot : Outport  Port=2
  J_CoM : Outport  Port=3
  J_rot_task : Outport  Port=4
  J_LHand : Outport  Port=5
  J_RHand : Outport  Port=6
  JDot_nu_LFoot : Outport  Port=7
  JDot_nu_RFoot : Outport  Port=8
  JDot_nu_CoM : Outport  Port=9
  JDot_nu_rot_task : Outport  Port=10
  JDot_nu_LHand : Outport  Port=11
  JDot_nu_RHand : Outport  Port=12
  wires:
  Jacobian CoM/1 -> J_CoM/1
  Jacobian rotational task/1 -> J_rot_task/1
  Jacobian LFoot/1 -> J_LFoot/1
  Jacobian RFoot/1 -> J_RFoot/1
  w_H_b/1 -> Jacobian rotational task/1, Jacobian RFoot1/1, Jacobian LFoot1/1, Jacobian CoM/1, Jacobian RFoot/1, Jacobian LFoot/1, DotJ Nu CoM/1, DotJ Nu LHand/1, DotJ Nu RHand/1, DotJ Nu rotational task/1, DotJ Nu Rfoot/1, DotJ Nu LFoot/1
  sDot/1 -> DotJ Nu LFoot/4, DotJ Nu Rfoot/4, DotJ Nu RHand/4, DotJ Nu LHand/4, DotJ Nu rotational task/4, DotJ Nu CoM/4
  nu_b/1 -> DotJ Nu LHand/3, DotJ Nu RHand/3, DotJ Nu LFoot/3, DotJ Nu Rfoot/3, DotJ Nu CoM/3, DotJ Nu rotational task/3
  s/1 -> Jacobian rotational task/2, Jacobian RFoot1/2, Jacobian LFoot1/2, Jacobian CoM/2, Jacobian RFoot/2, Jacobian LFoot/2, DotJ Nu CoM/2, DotJ Nu LHand/2, DotJ Nu RHand/2, DotJ Nu rotational task/2, DotJ Nu Rfoot/2, DotJ Nu LFoot/2
  DotJ Nu Rfoot/1 -> JDot_nu_RFoot/1
  DotJ Nu LFoot/1 -> JDot_nu_LFoot/1
  DotJ Nu rotational task/1 -> JDot_nu_rot_task/1
  DotJ Nu CoM/1 -> JDot_nu_CoM/1
  Jacobian RFoot1/1 -> J_RHand/1
  Jacobian LFoot1/1 -> J_LHand/1
  DotJ Nu LHand/1 -> JDot_nu_LHand/1
  DotJ Nu RHand/1 -> JDot_nu_RHand/1

== system torqueWalkingMultipleStateCoefficientR2017b/Dynamics and Kinematics/Inverse Kinematics/QP-Based Inverse Kinematics ==
  q_0 : Inport
  nu_0 : Inport  Port=2
  s_sDot_sDDot_ref : Inport  Port=3
  J : Inport  Port=4
  JDot_nu : Inport  Port=5
  acc_task_star : Inport  Port=6
  impedances : Inport  Port=7
  dampings : Inport  Port=8
  feetInContact : Inport  Port=9
  "Compute QP Hessian, gradient and constraints " : MATLAB Function  TreatAsAtomicUnit=on
  DoFs converter1 : WBToolboxLibrary/Utilities/DoFs converter  yarp2WBIOption=From YARP to WBI
      settings: SourceProductName=Whole Body Toolbox
  QP Solver (inverse kinematics) : Subsystem
  QP output : Scope  NumInputPorts=6
  Selector1 : Selector  InputPortWidth=ROBOT_DOF+6  IndexOptions=Index vector (dialog)  Indices=[7:29]  OutputSizes=1
  Selector3 : Selector  InputPortWidth=ROBOT_DOF+16  IndexOptions=Index vector (dialog)  Indices=[17:ROBOT_DOF+16]  OutputSizes=1
  inverse kinematics integration : Subsystem
  s_sDot_sDDot_des : Outport
  ExitFlagQP : Outport  Port=2
  nuDot : Outport  Port=3
  q : Outport  Port=4
  nu : Outport  Port=5
  wires:
  q_0/1 -> inverse kinematics integration/3(q_0)
  nu_0/1 -> inverse kinematics integration/2(nu_0)
  QP Solver (inverse kinematics)/1(nuDot) -> Selector1/1, inverse kinematics integration/1(nuDot), nuDot/1
  "Compute QP Hessian, gradient and constraints "/4(biasVectorConstraint) -> QP Solver (inverse kinematics)/4(biasVectorConstraint)
  "Compute QP Hessian, gradient and constraints "/3(ConstraintMatrix) -> QP Solver (inverse kinematics)/3(ConstraintMatrix)
  "Compute QP Hessian, gradient and constraints "/2(gradient) -> QP Solver (inverse kinematics)/2(gradient)
  "Compute QP Hessian, gradient and constraints "/1(Hessian) -> QP Solver (inverse kinematics)/1(Hessian)
  impedances/1 -> "Compute QP Hessian, gradient and constraints "/4(impedances)
  dampings/1 -> "Compute QP Hessian, gradient and constraints "/5(dampings)
  s_sDot_sDDot_ref/1 -> "Compute QP Hessian, gradient and constraints "/3(s_sDot_sDDot_ref)
  inverse kinematics integration/3(s_sDot_sDDot_des) -> s_sDot_sDDot_des/1
  inverse kinematics integration/2(q) -> q/1, Selector3/1
  Selector3/1 -> "Compute QP Hessian, gradient and constraints "/1(s)
  QP Solver (inverse kinematics)/2(ExitFlagQP) -> QP output/6, ExitFlagQP/1
  inverse kinematics integration/1(nu) -> nu/1, "Compute QP Hessian, gradient and constraints "/2(nu)
  J/1 -> "Compute QP Hessian, gradient and constraints "/6(J)
  JDot_nu/1 -> "Compute QP Hessian, gradient and constraints "/7(JDot_nu)
  acc_task_star/1 -> "Compute QP Hessian, gradient and constraints "/8(acc_task_star)
  feetInContact/1 -> "Compute QP Hessian, gradient and constraints "/9(feetInContact)
  Selector1/1 -> DoFs converter1/1
  DoFs converter1/1 -> QP output/1
  DoFs converter1/2 -> QP output/2
  DoFs converter1/3 -> QP output/3
  DoFs converter1/4 -> QP output/4
  DoFs converter1/5 -> QP output/5
